simulink model "pr725"  (R2018b)
settings: Solver=VariableStepAuto  StartTime=0.0  StopTime=200/Rb  RelTol=1e-3
PreLoadFcn:
  | Rb=1e6; % битовая скорость
libraries: commfilt2 x4, commrandsrc3 x1, commdigbbndpm3 x1
settings Model: Creator=Григорий Фокин  LastModifiedBy=Григорий Фокин

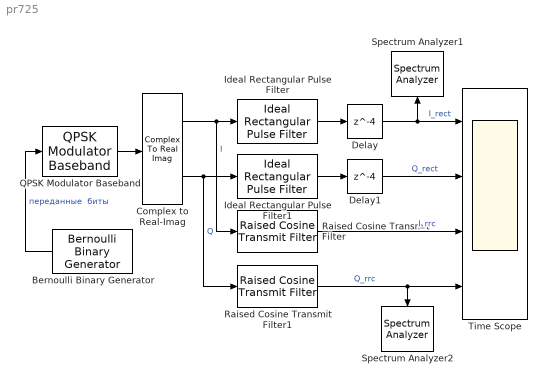
== system pr725 ==
  Bernoulli Binary Generator : commrandsrc3/Bernoulli Binary Generator  ProbabilityOfZero=0.5  SeedSource=Auto  Seed=0  SampleTime=1/Rb  SamplesPerFrame=2  OutputDataType=double  SimulateUsing=Interpreted execution
  Complex to Real-Imag : ComplexToRealImag
  Delay : Delay  DelayLength=4  InitialCondition=0
  Delay1 : Delay  DelayLength=4  InitialCondition=0
  Ideal Rectangular Pulse Filter : commfilt2/Ideal Rectangular Pulse Filter  pulseLen=8  pulseDelay=0  InputProcessing=Columns as channels (frame based)  RateOptions=Enforce single-rate processing  sampMode=Mute  normCheck=off  normMode=Sum of samples  filterGain=1  saveAsFlag=0  roundingMode=Floor  overflowMode=off  firstCoeffDataTypeStr=Inherit: Same word length as input  firstCoeffMin=[]  firstCoeffMax=[]  firstCoeffLastDataTypeStr=Inherit: Same word length as input  outputDataTypeStr=Inherit: Same as accumulator  outputMin=[]  outputMax=[]  outputLastDataTypeStr=Inherit: Same as accumulator
      settings: SourceProductName=Communications System Toolbox  SourceProductBaseCode=CM
  Ideal Rectangular Pulse Filter1 : commfilt2/Ideal Rectangular Pulse Filter  pulseLen=8  pulseDelay=0  InputProcessing=Columns as channels (frame based)  RateOptions=Enforce single-rate processing  sampMode=Mute  normCheck=off  normMode=Sum of samples  filterGain=1  saveAsFlag=0  roundingMode=Floor  overflowMode=off  firstCoeffDataTypeStr=Inherit: Same word length as input  firstCoeffMin=[]  firstCoeffMax=[]  firstCoeffLastDataTypeStr=Inherit: Same word length as input  outputDataTypeStr=Inherit: Same as accumulator  outputMin=[]  outputMax=[]  outputLastDataTypeStr=Inherit: Same as accumulator
      settings: SourceProductName=Communications System Toolbox  SourceProductBaseCode=CM
  QPSK Modulator Baseband : commdigbbndpm3/QPSK Modulator Baseband  InType=Bit  Enc=Gray  Ph=pi/4  outDtype=double  outWordLen=16  outUDDataType=sfix(16)  outFracLenMode=Best precision  outFracLen=15  outDataTypeStr=double  outLastDataTypeStr=double
  Raised Cosine Transmit Filter : commfilt2/Raised Cosine Transmit Filter  filtType=Square root  R=0.2  filtSpan=10  N=8  filterGain=1  InputProcessing=Columns as channels (frame based)  RateOptions=Enforce single-rate processing  framing=Mute  checkCoeff=off  variableName=rcTxFilt  checkGain=Normalized  sampMode=Mute  saveAsFlag=0  currentFiltSpan=10  D=(10)/2  launchFVT=on  roundingMode=Floor  overflowMode=off  coeffDataTypeStr=Inherit: Same word length as input  coeffMin=[]  coeffMax=[]  coeffLastDataTypeStr=Inherit: Same word length as input  outputDataTypeStr=Inherit: Same as accumulator  outputMin=[]  outputMax=[]  outputLastDataTypeStr=Inherit: Same as accumulator
  Raised Cosine Transmit Filter1 : commfilt2/Raised Cosine Transmit Filter  filtType=Square root  R=0.2  filtSpan=10  N=8  filterGain=1  InputProcessing=Columns as channels (frame based)  RateOptions=Enforce single-rate processing  framing=Mute  checkCoeff=off  variableName=rcTxFilt1  checkGain=Normalized  sampMode=Mute  saveAsFlag=0  currentFiltSpan=10  D=(10)/2  launchFVT=on  roundingMode=Floor  overflowMode=off  coeffDataTypeStr=Inherit: Same word length as input  coeffMin=[]  coeffMax=[]  coeffLastDataTypeStr=Inherit: Same word length as input  outputDataTypeStr=Inherit: Same as accumulator  outputMin=[]  outputMax=[]  outputLastDataTypeStr=Inherit: Same as accumulator
  Spectrum Analyzer1 : SpectrumAnalyzer
  Spectrum Analyzer2 : SpectrumAnalyzer
  Time Scope : Scope  NumInputPorts=4
  wires:
  Bernoulli Binary Generator/1 -> QPSK Modulator Baseband/1  "переданные  биты"
  QPSK Modulator Baseband/1 -> Complex to Real-Imag/1
  Complex to Real-Imag/1 -> Ideal Rectangular Pulse Filter/1, Raised Cosine Transmit Filter/1  "I"
  Complex to Real-Imag/2 -> Raised Cosine Transmit Filter1/1, Ideal Rectangular Pulse Filter1/1  "Q"
  Ideal Rectangular Pulse Filter/1 -> Delay/1
  Ideal Rectangular Pulse Filter1/1 -> Delay1/1
  Raised Cosine Transmit Filter/1 -> Time Scope/3  "I_rrc"
  Raised Cosine Transmit Filter1/1 -> Spectrum Analyzer2/1, Time Scope/4  "Q_rrc"
  Delay/1 -> Time Scope/1, Spectrum Analyzer1/1  "I_rect"
  Delay1/1 -> Time Scope/2  "Q_rect"
